simulink model "SistemaControlo_Sem_pert_atuador"  (R2018b)
settings: Solver=VariableStepAuto  StartTime=0.0  StopTime=600  RelTol=1e-3
libraries: fuzblock x1
settings Model: SimulationMode=accelerator  Creator=novo  LastModifiedBy=Principe
settings SolverCC: ZeroCrossAlgorithm=Adaptive
settings SFSimCC: SimUseLocalCustomCode=off
settings RTWCC: RTWUseLocalCustomCode=off
settings CodeAppCC: StateflowObjectComments=on

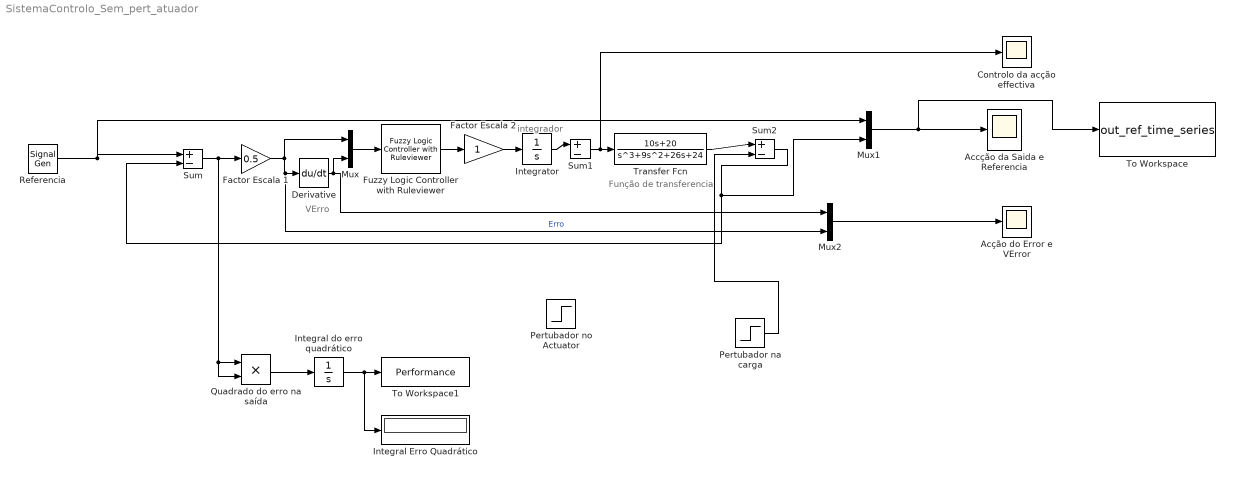
== system SistemaControlo_Sem_pert_atuador ==
  note: Função de transferencia
  note: integrador
  note: VErro
  Accção da Saida e Referencia : Scope
  Acção do Error e VError : Scope
  Controlo da acção effectiva : Scope
  Derivative : Derivative
  Factor Escala 1 : Gain  Gain=0.5
  Factor Escala 2 : Gain
  Fuzzy Logic Controller with Ruleviewer : fuzblock/Fuzzy Logic  Controller  with Ruleviewer  fismatrix=sug25  Ts=4
  Integral Erro Quadrático : Display
  Integral do erro quadrático : Integrator
  Integrator : Integrator
  Mux : Mux  Inputs=2
  Mux1 : Mux  Inputs=2
  Mux2 : Mux  Inputs=2
  Pertubador na carga : Step  Time=190  SampleTime=0
  Pertubador no Actuator : Step  Time=100  SampleTime=0
  Quadrado do erro na saída : Product
  Referencia : SignalGenerator  Frequency=0.1  Units=rad/sec
  Sum : Sum  Inputs=|+-
  Sum1 : Sum  Inputs=|+-
  Sum2 : Sum  Inputs=|+-
  To Workspace : ToWorkspace  VariableName=out_ref_time_series  SaveFormat=Timeseries  SampleTime=-1
  To Workspace1 : ToWorkspace  VariableName=Performance  SaveFormat=Timeseries  SampleTime=-1
  Transfer Fcn : TransferFcn  Numerator=[10 20]  Denominator=[1 9 26 24]
  wires:
  Referencia/1 -> Sum/1, Mux1/1
  Factor Escala 1/1 -> Mux/1, Mux2/2, Derivative/1  "Erro"
  Derivative/1 -> Mux2/1, Mux/2
  Mux/1 -> Fuzzy Logic Controller with Ruleviewer/1
  Factor Escala 2/1 -> Integrator/1
  Fuzzy Logic Controller with Ruleviewer/1 -> Factor Escala 2/1
  Integrator/1 -> Sum1/1
  Sum1/1 -> Controlo da acção effectiva/1, Transfer Fcn/1
  Transfer Fcn/1 -> Sum2/1
  Sum2/1 -> Mux1/2, Sum/2
  Pertubador na carga/1 -> Sum2/2
  Mux2/1 -> Acção do Error e VError/1
  Mux1/1 -> To Workspace/1, Accção da Saida e Referencia/1
  Integral do erro quadrático/1 -> Integral Erro Quadrático/1, To Workspace1/1
  Sum/1 -> Quadrado do erro na saída/2, Quadrado do erro na saída/1, Factor Escala 1/1
  Quadrado do erro na saída/1 -> Integral do erro quadrático/1
